simulink model "SimulinkOfTheProject"  (R2016a)
settings: Solver=VariableStepAuto  SolverMode=SingleTasking  StartTime=0.0  StopTime=10.0  RelTol=1e-3
settings Model: Creator=Kasra  LastModifiedBy=Kasra
settings DebuggingCC: SFUnexpectedBacktrackingDiag=error  SFNoUnconditionalDefaultTransitionDiag=error
settings GRTTargetCC: TargetLangStandard=C99 (ISO)  GeneratePreprocessorConditionals=Use local settings
settings ConfigComp: CovMetricSettings=dwe  CovHtmlReporting=off  CovSaveCumulativeToWorkspaceVar=off  CovSaveSingleToWorkspaceVar=off  CovExternalEMLEnable=on

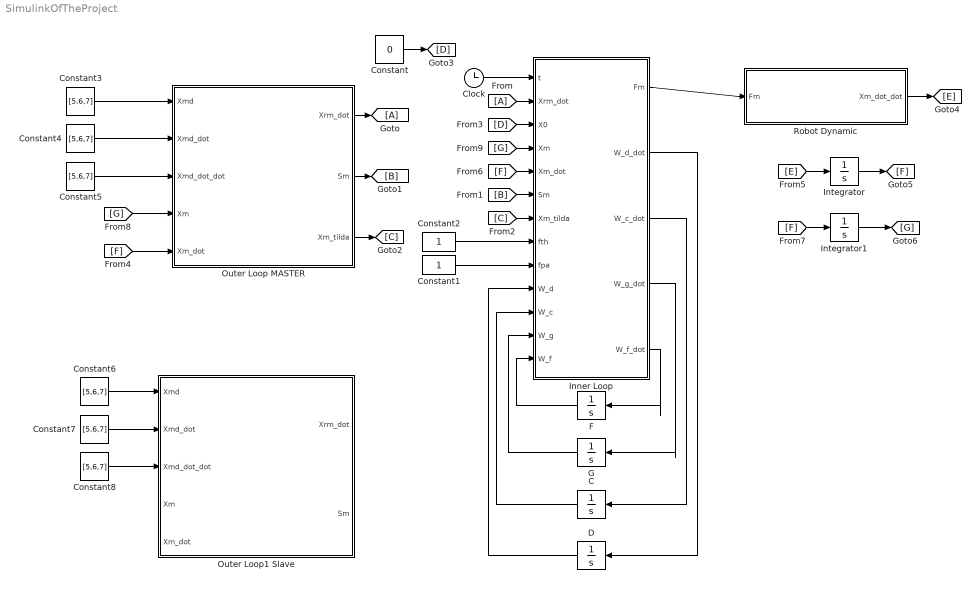
== system SimulinkOfTheProject ==
  C : Integrator
  Clock : Clock
  Constant : Constant  Value=0
  Constant1 : Constant
  Constant2 : Constant
  Constant{3..8} (6 alike) : Constant  Value=[5,6,7]
  D : Integrator
  F : Integrator
  G : Integrator
  Inner Loop : MATLAB Function  TreatAsAtomicUnit=on
  Integrator : Integrator
  Integrator1 : Integrator
  Outer Loop MASTER : MATLAB Function  TreatAsAtomicUnit=on
  Outer Loop1 Slave : MATLAB Function  TreatAsAtomicUnit=on
  Robot Dynamic : MATLAB Function  TreatAsAtomicUnit=on
  wires:
  Inner Loop/4(W_g_dot) -> G/1
  G/1 -> Inner Loop/12(W_g)
  Inner Loop/3(W_c_dot) -> C/1
  C/1 -> Inner Loop/11(W_c)
  Inner Loop/2(W_d_dot) -> D/1
  D/1 -> Inner Loop/10(W_d)
  Clock/1 -> Inner Loop/1(t)
  Inner Loop/1(Fm) -> Robot Dynamic/1(Fm)
  Inner Loop/5(W_f_dot) -> F/1
  F/1 -> Inner Loop/13(W_f)
  [A] -> Inner Loop/2(Xrm_dot)
  Outer Loop MASTER/1(Xrm_dot) -> [A]
  [B] -> Inner Loop/6(Sm)
  Outer Loop MASTER/2(Sm) -> [B]
  [C] -> Inner Loop/7(Xm_tilda)
  Outer Loop MASTER/3(Xm_tilda) -> [C]
  [D] -> Inner Loop/3(X0)
  Constant/1 -> [D]
  Robot Dynamic/1(Xm_dot_dot) -> [E]
  [E] -> Integrator/1
  [F] -> Outer Loop MASTER/5(Xm_dot)
  [F] -> Inner Loop/5(Xm_dot)
  [F] -> Integrator1/1
  Integrator/1 -> [F]
  Integrator1/1 -> [G]
  [G] -> Outer Loop MASTER/4(Xm)
  [G] -> Inner Loop/4(Xm)
  Constant1/1 -> Inner Loop/9(fpa)
  Constant2/1 -> Inner Loop/8(fth)
  Constant3/1 -> Outer Loop MASTER/1(Xmd)
  Constant5/1 -> Outer Loop MASTER/3(Xmd_dot_dot)
  Constant4/1 -> Outer Loop MASTER/2(Xmd_dot)
  Constant6/1 -> Outer Loop1 Slave/1(Xmd)
  Constant7/1 -> Outer Loop1 Slave/2(Xmd_dot)
  Constant8/1 -> Outer Loop1 Slave/3(Xmd_dot_dot)

== matlab function SimulinkOfTheProject/Robot Dynamic ==
  data: Fm input; Xm_dot_dot output
function Xm_dot_dot = fcn(Fm)

Xm_dot_dot = Fm;

== matlab function SimulinkOfTheProject/Inner Loop ==
  data: t input; Xrm_dot input; X0 input; Xm input; Xm_dot input; Sm input; Xm_tilda input; fth input; fpa input; Fm output; W_d_dot output; W_c_dot output; W_g_dot output; W_d input; W_c input; W_g input; W_f_dot output; W_f input
function [Fm, W_d_dot, W_c_dot, W_g_dot, W_f_dot]= fcn(t, Xrm_dot, X0, Xm, Xm_dot, Sm, Xm_tilda, fth, fpa, W_d, W_c, W_g, W_f)

fn = 50;
Kf = 0.5;
Mm = 1;
lambda3m = 2;
Xm_tilda = Xmod - Xm;

zz = [1;sin(fn*t);sin(2*fn*t)];

Zd = [zz, zeros(6, 1); zeros(3, 1), zz, zeros(3, 1); zeros(6, 1), zz];
Zc = Zd;
Zg = zz;
Zf = zz;

D_hat = W_d' * Zd;
C_hat = W_c' * Zc;
g_hat = W_g' * Zg;
f_hat = W_f' * Zf;

Qd = 100 * eye(9);
Qc = 100 * eye(9);
Qg = 100 * eye(3);
Qf = 100 * eye(3);

P = -(pinv(Mm)*Cm)*Xm_dot - (pinv(Mm)*Km)*(Xm-X0) + pinv(Mm)*(fth-Kf*fpa) + ((lambda3m)^2)*Xm_tilda;
Fm = D_hat * P + C_hat * Xrm_dot + g_hat + f_hat;

W_d_dot = (Sm*P*(Zd')*pinv(Qd))';
W_c_dot = (Sm*(Xrm_dot')*(Zc')*pinv(Qc))';
W_g_dot = (Sm*(Zg')*pinv(Qg))';
W_f_dot = (Sm*(Zf')*pinv(Qf))';

== matlab function SimulinkOfTheProject/Outer Loop MASTER ==
  data: Xmd input; Xrm_dot output; Sm output; Xmd_dot input; Xmd_dot_dot input; Xm input; Xm_dot input; Xm_tilda output
function [Xrm_dot, Sm, Xm_tilda] = fcn(Xmd, Xmd_dot, Xmd_dot_dot, Xm, Xm_dot)
l1 = 1;
Xrm_dot = Xmd_dot - l1 * (Xm - Xmd);
Sm = Xm_dot - Xrm_dot;
Xm_tilda = Xmd-Xm;

== matlab function SimulinkOfTheProject/Outer Loop1 Slave ==
  data: Xmd input; Xrm_dot output; Sm output; Xmd_dot input; Xmd_dot_dot input; Xm input; Xm_dot input
function [Xrm_dot, Sm] = fcn(Xmd, Xmd_dot, Xmd_dot_dot, Xm, Xm_dot)
l1 = 1;
Xrm_dot = Xmd_dot - l1 * (Xm - Xmd);
Sm = Xm_dot - Xrm_dot;
